simulink model "mass_damper"  (R2022b)
settings: Solver=VariableStepAuto  StartTime=0.0  StopTime=50  RelTol=1e-3
settings Model: Creator=dangm  LastModifiedBy=ASUS
settings SolverCC: AlgebraicLoopSolver=TrustRegion
settings DebuggingCC: UnconnectedInputMsg=warning  UnconnectedOutputMsg=warning  UnconnectedLineMsg=warning  SFMachineParentedDataDiag=warning
settings ModelReferenceCC: EnableRefExpFcnMdlSchedulingChecks=on

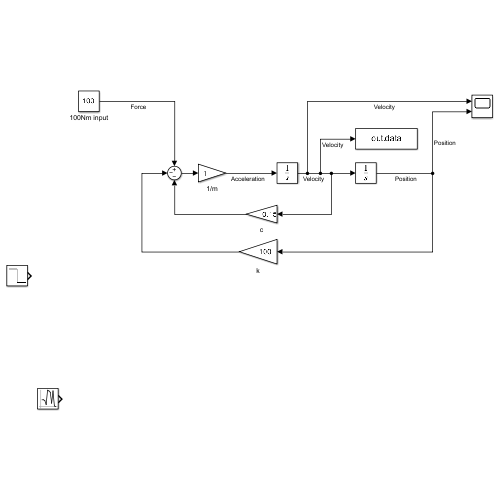
[thumbnail: Simulink's stored preview of the top-level diagram]
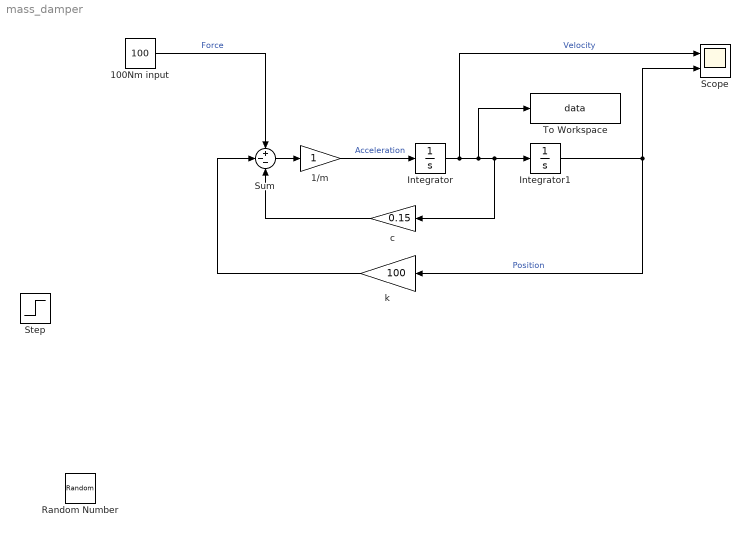
== system mass_damper ==
  1/m : Gain
  100Nm input : Constant  Value=100
  Integrator : Integrator
  Integrator1 : Integrator
  Random Number : RandomNumber  Variance=100  SampleTime=0.1
  Scope : Scope  NumInputPorts=2
  Step : Step  Time=0.1  Before=1  After=0  SampleTime=0
  Sum : Sum  Inputs=+--
  To Workspace : ToWorkspace  VariableName=data  SaveFormat=Timeseries  SampleTime=-1
  c : Gain  Gain=0.15
  k : Gain  Gain=100
  wires:
  Integrator/1 -> Scope/1, To Workspace/1, c/1, Integrator1/1  "Velocity"
  Sum/1 -> 1/m/1
  Integrator1/1 -> k/1, Scope/2  "Position"
  k/1 -> Sum/2
  1/m/1 -> Integrator/1  "Acceleration"
  c/1 -> Sum/3
  100Nm input/1 -> Sum/1  "Force"
